simulink library "tqd"  (R2021b)
settings: Solver=VariableStepAuto  StartTime=0.0  StopTime=10.0  RelTol=1e-3
undefined symbols (not defined in the file or in its folder): ATQD_APSDecReq_X_kph, ATQD_APSDecReq_Y_mps2, ATQD_APSDecReqCMD_X_kph, ATQD_APSDecReqTs_X_pct, ATQD_APSDecTimeGain_X_Deg, ATQD_APSDecTimeGain_Y_s, ATQD_APSReqLowSpd_X_Deg, ATQD_AutoHoldReleaseBPS_X_Deg, ATQD_AWDLoadTrqnsGain_X_kg, ATQD_AWDLoadTrqnsGain_Y_pct, ATQD_BOSEnBPSPosn_X_kph, ATQD_BOSMap_X_rpm, ATQD_BOSMap_Y_pct, ATQD_CreepBaseTqD_X_kph, ATQD_CreepBaseTqD_Y_Deg, ATQD_CreepBaseTqR_X_kph, ATQD_CreepBaseTqR_Y_Deg, ATQD_CreepBPSDisPosn_X_Deg, ATQD_CreepBPSDisPosnR_X_Deg, ATQD_CreepBPSEnPosn_X_Deg, ATQD_CreepBPSEnPosnR_X_Deg, ATQD_CreepDeltaTq_X_kph, ATQD_CreepIterm_X_kph, ATQD_CreepIterm_Y_kph, ATQD_CreepItermMaxLimit_X_pct, ATQD_CreepPreloadTime_X_kph, ATQD_CreepPreloadTq_X_kph, ATQD_CreepPreloadTq_Y_s, ATQD_CreepProtTq_X_Deg, ATQD_CreepPterm_X_kph, ATQD_ECOTqMapD_X_rpm, ATQD_ECOTqMapD_Y_pct, ATQD_EOPDTqMapDCon_X_rpm, ATQD_EOPDTqMapDCon_Y_Deg, ATQD_EstInitVehWeight_X_c, ATQD_LHMRollGenMapD_X_rpm, ATQD_LHMRollGenMapD_Y_rpm, ATQD_LHMTqMapD_X_rpm, ATQD_LHMTqMapD_Y_pct, ATQD_NL1TqMapD_X_rpm, ATQD_NL1TqMapD_Y_pct, ATQD_NOPDTqMapDCon_X_rpm, ATQD_NOPDTqMapDCon_Y_Deg, ATQD_NRMRrEDUSpRat_X_rpm, ATQD_NRMRrEDUSpRat_Y_Nm, ATQD_OPDHoldDownRelDelay_X_Deg, ATQD_OPDHoldEnSpd_X_Deg, ATQD_OPDHoldRelDetTime_X_Deg, ATQD_OPDHoldReleaseTq_X_Deg, ATQD_OrigPedTqLowLim_X_Deg, ATQD_OrigPedTqLowLim_Y_pct, ATQD_PedalMapClimbUpLim_X_rpm, ATQD_PedalMapClimbUpLim_Y_Deg, ATQD_PreLoadTq_X_s, ATQD_RollGenMapEL1_X_rpm, ATQD_RollGenMapEL1_Y_rpm, ATQD_SL1TqMapD_X_rpm, ATQD_SL1TqMapD_Y_pct, ATQD_SlideRegenTqGain_X_Gps, ATQD_SlideRegenTqGain_Y_pct ... (+444)
libraries: hcu_lib x70, simulink x61, tqr x1
(part 3 of 14)

== system tqd/TQD/TorqueDemand/ShiftModule ==
  task_time_s : Inport
  VINP_ShifterHandleCmd_enum : Inport  Port=2
  VINP_VehSpeed_kph : Inport  Port=3
  VTQD_BrkSwSta_flg : Inport  Port=4
  VPMM_PowerSta_enum : Inport  Port=5
  VINP_PBWMotorPos_enum : Inport  Port=6
  VTQD_TMRotateDirction_enum : Inport  Port=7
  VTQD_EPBCarWashMode_flg : Inport  Port=8
  VINP_DrDoorSW_flg : Inport  Port=9
  VVMC_APSShiftPosnReq_enum : Inport  Port=10
  VVMC_APSActive_flg : Inport  Port=11
  VINP_DriverSeatBeltCmd_flg : Inport  Port=12
  VINP_SeatSW_flg : Inport  Port=13
  VINP_ChrgPlugSta_enum : Inport  Port=14
  VTQD_IVIPwrLock_flg : Inport  Port=15
  VTQD_AfterAvailableTqDemFr_Nm : Inport  Port=16
  VTQD_AfterAvailableTqDemRr_Nm : Inport  Port=17
  VTQR_NoABSFEDUWhlTqReq_Nm : Inport  Port=18
  VTQR_NoABSREDUWhlTqReq_Nm : Inport  Port=19
  VINP_DOASta_flg : Inport  Port=20
  VINP_MCPressure_bar : Inport  Port=21
  VTQD_OPDHoldAllowPark_flg : Inport  Port=22
  Constant : Constant  Value=KTQD_VehSpd2P_kph
  Constant1 : Constant  Value=KTQD_PBWTimeout_s
  Constant2 : Constant  Value=KTQD_VehSpdRev_kph
  Constant3 : Constant  Value=KTQD_ShiftInitialTime_s
  Constant4 : Constant  Value=KTQD_RelockWaitTime_s
  Constant5 : Constant  Value=KTQD_ReunlockWaitTime_s
  Constant6 : Constant  Value=ENUM_GEARACTUALPOSN_P
  Constant7 : Constant  Value=ENUM_GEARACTUALPOSN_P
  Data Type Conversion1 : DataTypeConversion
  Data Type Conversion2 : DataTypeConversion
  Data Type Conversion3 : DataTypeConversion  OutDataTypeStr=uint8
  Data Type Conversion4 : DataTypeConversion  OutDataTypeStr=boolean
  Determine_Actual_Gear_Position : Stateflow chart  TreatAsAtomicUnit=on
  Equal : RelationalOperator  Operator===  OutDataTypeStr=boolean  RndMeth=Simplest
  Equal1 : RelationalOperator  Operator=~=  OutDataTypeStr=boolean  RndMeth=Simplest
  GearShiftPosn : Subsystem  Description=GearPosition
  P_Button_State_Judge : Subsystem
  SR_Latch : hcu_lib/Basic_Blocks/SR_Latch
  SR_Latch1 : Subsystem  mask(SR_Latch){}
      mask help: SR latch function.
  VTQD_GearActualPosn_enum : Outport
  VTQD_ParkRequest_flg : Outport  Port=2
  VTQD_PBWLockTO_flg : Outport  Port=3
  VTQD_PBWUnlockTO_flg : Outport  Port=4
  VTQD_PButtonSta_enum : Outport  Port=5
  VTQD_DriveProtRemove_flg : Outport  Port=6
  VTQD_DriveProtEn_flg : Outport  Port=7
  wires:
  VPMM_PowerSta_enum/1 -> [VPMM_PowerSta_enum]
  task_time_s/1 -> [task_time_s]
  VINP_VehSpeed_kph/1 -> [VINP_VehSpeed_kph]
  VTQD_BrkSwSta_flg/1 -> [VTQD_BrkSwSta_flg]
  VTQD_TMRotateDirction_enum/1 -> [VTQD_TMRotateDirction_enum]
  VINP_PBWMotorPos_enum/1 -> [VINP_PBWMotorPos_enum]
  P_Button_State_Judge/1(VTQD_PButtonSta_enum) -> VTQD_PButtonSta_enum/1
  VINP_ShifterHandleCmd_enum/1 -> [VINP_ShifterHandleCmd_enum]
  [VINP_ShifterHandleCmd_enum] -> P_Button_State_Judge/1(VINP_ShifterHandleCmd_enum)
  VTQD_IVIPwrLock_flg/1 -> [VTQD_IVIPwrLock_flg]
  VINP_ChrgPlugSta_enum/1 -> [VINP_ChrgPlugSta_enum]
  VINP_SeatSW_flg/1 -> [VINP_SeatSW_flg]
  VINP_DriverSeatBeltCmd_flg/1 -> [VINP_DriverSeatBeltCmd_flg]
  VVMC_APSActive_flg/1 -> [VVMC_APSActive_flg]
  VVMC_APSShiftPosnReq_enum/1 -> [VVMC_APSShiftPosnReq_enum]
  VINP_DrDoorSW_flg/1 -> [VINP_DrDoorSW_flg]
  VTQD_EPBCarWashMode_flg/1 -> [VTQD_EPBCarWashMode_flg]
  [VTQD_EPBCarWashMode_flg] -> GearShiftPosn/8(VTQD_EPBCarWashMode_flg)
  [VINP_VehSpeed_kph] -> GearShiftPosn/9(VINP_VehSpeed_kph)
  [VINP_ChrgPlugSta_enum] -> GearShiftPosn/10(VINP_ChrgPlugSta_enum)
  GearShiftPosn/3(VTQD_PwrStaAllowDR_flg) -> [VTQD_PwrStaAllowDR_flg]
  [VVMC_APSShiftPosnReq_enum] -> GearShiftPosn/4(VVMC_APSShiftPosnReq_enum)
  [VINP_DrDoorSW_flg] -> GearShiftPosn/3(VINP_DrDoorSW_flg)
  [VINP_ShifterHandleCmd_enum] -> GearShiftPosn/1(VINP_ShifterHandleCmd_enum)
  [VVMC_APSActive_flg] -> GearShiftPosn/5(VVMC_APSActive_flg)
  [VINP_DriverSeatBeltCmd_flg] -> GearShiftPosn/6(VINP_DriverSeatBeltCmd_flg)
  GearShiftPosn/1(VTQD_GearShiftCMD_enum) -> [VTQD_GearShiftCMD_enum]
  [VINP_SeatSW_flg] -> GearShiftPosn/7(VINP_SeatSW_flg)
  [VPMM_PowerSta_enum] -> GearShiftPosn/2(VPMM_PowerSta_enum)
  GearShiftPosn/2(VTQD_PwrStaAllowPN_flg) -> [VTQD_PwrStaAllowPN_flg]
  [VVMC_APSActive_flg] -> Determine_Actual_Gear_Position/16(VVMC_APSActive_flg)
  Data Type Conversion4/1 -> VTQD_ParkRequest_flg/1  "VTQD_ParkRequest_flg"
  Constant6/1 -> Equal/2
  [VTQD_EPBCarWashMode_flg] -> Determine_Actual_Gear_Position/15(VINP_EPBCarWashMode_flg)
  Constant4/1 -> Determine_Actual_Gear_Position/13(KTQD_RelockWaitTime_s)
  Constant2/1 -> Determine_Actual_Gear_Position/10(KTQD_VehSpdRev_kph)
  Data Type Conversion1/1 -> SR_Latch/1
  [VTQD_GearActualPosn_enum] -> Equal1/1
  [VTQD_GearActualPosn_enum] -> Equal/1
  Data Type Conversion2/1 -> SR_Latch1/1(set)
  Determine_Actual_Gear_Position/4(VTQD_ParkRequest_flg) -> Data Type Conversion4/1
  Constant7/1 -> Equal1/2
  Data Type Conversion3/1 -> [VTQD_GearActualPosn_enum], VTQD_GearActualPosn_enum/1  "VTQD_GearActualPosn_enum"
  Constant1/1 -> Determine_Actual_Gear_Position/12(KTQD_PBWTimeout_s)
  Constant5/1 -> Determine_Actual_Gear_Position/14(KTQD_ReunlockWaitTime_s)
  [VTQD_PwrStaAllowPN_flg] -> Determine_Actual_Gear_Position/7(VTQD_PwrStaAllowPN_flg)
  Determine_Actual_Gear_Position/3(VTQD_PBWUnlockTO_flg) -> Data Type Conversion2/1
  Constant/1 -> Determine_Actual_Gear_Position/9(KTQD_VehSpd2P_kph)
  [VTQD_TMRotateDirction_enum] -> Determine_Actual_Gear_Position/8(VTQD_TMRotateDirction_enum)
  SR_Latch1/1(latched) -> VTQD_PBWUnlockTO_flg/1  "VTQD_PBWUnlockTO_flg"
  Equal1/1 -> SR_Latch1/2(reset)
  [VINP_VehSpeed_kph] -> Determine_Actual_Gear_Position/4(VINP_VehSpd_kph)
  [VTQD_PwrStaAllowDR_flg] -> Determine_Actual_Gear_Position/6(VTQD_PwrStaAllowDR_flg)
  Constant3/1 -> Determine_Actual_Gear_Position/11(KTQD_ShiftInitialTime_s)
  [VTQD_GearShiftCMD_enum] -> Determine_Actual_Gear_Position/3(VTQD_GearShiftCMD_enum)
  Equal/1 -> SR_Latch/2
  [task_time_s] -> Determine_Actual_Gear_Position/1(task_time_s)
  [VTQD_BrkSwSta_flg] -> Determine_Actual_Gear_Position/2(VTQD_BrkSwSta_flg)
  Determine_Actual_Gear_Position/2(VTQD_PBWLockTO_flg) -> Data Type Conversion1/1
  Determine_Actual_Gear_Position/1(VTQD_GearActualPosn_enum) -> Data Type Conversion3/1
  [VINP_PBWMotorPos_enum] -> Determine_Actual_Gear_Position/5(VINP_PBWMotorPos_enum)
  SR_Latch/1 -> VTQD_PBWLockTO_flg/1  "VTQD_PBWLockTO_flg"
  [VTQD_GearActualPosn_enum] -> GearShiftPosn/11(VTQD_GearActualPosn_enum)
  [VTQD_AfterAvailableTqDemFr_Nm] -> GearShiftPosn/12(VTQD_AfterAvailableTqDemFr_Nm)
  [VTQR_NoABSREDUWhlTqReq_Nm] -> GearShiftPosn/15(VTQR_NoABSREDUWhlTqReq_Nm)
  [VTQR_NoABSFEDUWhlTqReq_Nm] -> GearShiftPosn/14(VTQR_NoABSFEDUWhlTqReq_Nm)
  [VTQD_AfterAvailableTqDemRr_Nm] -> GearShiftPosn/13(VTQD_AfterAvailableTqDemRr_Nm)
  [task_time_s] -> GearShiftPosn/16(task_time_s)
  VTQD_AfterAvailableTqDemFr_Nm/1 -> [VTQD_AfterAvailableTqDemFr_Nm]
  VTQD_AfterAvailableTqDemRr_Nm/1 -> [VTQD_AfterAvailableTqDemRr_Nm]
  VTQR_NoABSFEDUWhlTqReq_Nm/1 -> [VTQR_NoABSFEDUWhlTqReq_Nm]
  VTQR_NoABSREDUWhlTqReq_Nm/1 -> [VTQR_NoABSREDUWhlTqReq_Nm]
  VINP_DOASta_flg/1 -> [VINP_DOASta_flg]
  [VINP_DOASta_flg] -> GearShiftPosn/17(VINP_DOASta_flg)
  GearShiftPosn/4(VTQD_DriveProtRemove_flg) -> VTQD_DriveProtRemove_flg/1
  GearShiftPosn/5(VTQD_DriveProtEn_flg) -> VTQD_DriveProtEn_flg/1
  [VTQD_IVIPwrLock_flg] -> GearShiftPosn/18(VTQD_IVIPwrLock_flg)
  [VTQD_BrkSwSta_flg] -> GearShiftPosn/19(VTQD_BrkSwSta_flg)
  GearShiftPosn/6(VTQD_ForceP_flg) -> [VTQD_ForceP_flg]
  [VTQD_ForceP_flg] -> Determine_Actual_Gear_Position/17(VTQD_ForceP_flg)
  VINP_MCPressure_bar/1 -> [VINP_MCPressure_bar]
  VTQD_OPDHoldAllowPark_flg/1 -> [VTQD_OPDHoldAllowPark_flg]
  [VTQD_OPDHoldAllowPark_flg] -> GearShiftPosn/20(VTQD_OPDHoldAllowPark_flg)
